simulink model "gm_parallel_lht_vnl"  (R2019b)
settings: Solver=FixedStepDiscrete  StartTime=0.0  StopTime=inf  RelTol=1e-3
undefined symbols (not defined in the file or in its folder): bt, height, nTheta, width
libraries: hdlsllib x199, simulink x27, hdlmdlgenlib x7, dspsrcs4 x1
(part 19 of 19)

== system gm_parallel_lht_vnl/Parallel LHT/Parallel LHT Kernel/Hough Kernel/Hough Kernel Symmetric Look Ahead/Look Ahead Hough/Register Bank_instance85 ==
  Data In : Inport  OutDataTypeStr=fixdt(1, 11, 0)  PortDimensions=1  SampleTime=6.66666666666667e-09
  Write Enable : Inport  Port=2  OutDataTypeStr=boolean  PortDimensions=1  SampleTime=6.66666666666667e-09
  Delay_Switch : Switch  Criteria=u2 ~= 0  Threshold=double(0)  OutDataTypeStr=fixdt(1, 11, 0)  SampleTime=6.66666666666667e-09
  Unit Delay Enabled Synchronous_lowered : Delay  DelayLength=double(1)  InitialCondition=0  SampleTime=6.66666666666667e-09
  Data Out : Outport
  wires:
  Unit Delay Enabled Synchronous_lowered/1 -> Data Out/1, Delay_Switch/3
  Data In/1 -> Delay_Switch/1
  Write Enable/1 -> Delay_Switch/2
  Delay_Switch/1 -> Unit Delay Enabled Synchronous_lowered/1

== system gm_parallel_lht_vnl/Parallel LHT/Parallel LHT Kernel/Hough Kernel/Hough Kernel Symmetric Look Ahead/Look Ahead Hough/Register Bank_instance86 ==
  Data In : Inport  OutDataTypeStr=fixdt(1, 11, 0)  PortDimensions=1  SampleTime=6.66666666666667e-09
  Write Enable : Inport  Port=2  OutDataTypeStr=boolean  PortDimensions=1  SampleTime=6.66666666666667e-09
  Delay_Switch : Switch  Criteria=u2 ~= 0  Threshold=double(0)  OutDataTypeStr=fixdt(1, 11, 0)  SampleTime=6.66666666666667e-09
  Unit Delay Enabled Synchronous_lowered : Delay  DelayLength=double(1)  InitialCondition=0  SampleTime=6.66666666666667e-09
  Data Out : Outport
  wires:
  Unit Delay Enabled Synchronous_lowered/1 -> Data Out/1, Delay_Switch/3
  Data In/1 -> Delay_Switch/1
  Write Enable/1 -> Delay_Switch/2
  Delay_Switch/1 -> Unit Delay Enabled Synchronous_lowered/1

== system gm_parallel_lht_vnl/Parallel LHT/Parallel LHT Kernel/Hough Kernel/Hough Kernel Symmetric Look Ahead/Look Ahead Hough/Register Bank_instance87 ==
  Data In : Inport  OutDataTypeStr=fixdt(1, 11, 0)  PortDimensions=1  SampleTime=6.66666666666667e-09
  Write Enable : Inport  Port=2  OutDataTypeStr=boolean  PortDimensions=1  SampleTime=6.66666666666667e-09
  Delay_Switch : Switch  Criteria=u2 ~= 0  Threshold=double(0)  OutDataTypeStr=fixdt(1, 11, 0)  SampleTime=6.66666666666667e-09
  Unit Delay Enabled Synchronous_lowered : Delay  DelayLength=double(1)  InitialCondition=0  SampleTime=6.66666666666667e-09
  Data Out : Outport
  wires:
  Unit Delay Enabled Synchronous_lowered/1 -> Data Out/1, Delay_Switch/3
  Data In/1 -> Delay_Switch/1
  Write Enable/1 -> Delay_Switch/2
  Delay_Switch/1 -> Unit Delay Enabled Synchronous_lowered/1

== system gm_parallel_lht_vnl/Parallel LHT/Parallel LHT Kernel/Hough Kernel/Hough Kernel Symmetric Look Ahead/Look Ahead Hough/Register Bank_instance88 ==
  Data In : Inport  OutDataTypeStr=fixdt(1, 11, 0)  PortDimensions=1  SampleTime=6.66666666666667e-09
  Write Enable : Inport  Port=2  OutDataTypeStr=boolean  PortDimensions=1  SampleTime=6.66666666666667e-09
  Delay_Switch : Switch  Criteria=u2 ~= 0  Threshold=double(0)  OutDataTypeStr=fixdt(1, 11, 0)  SampleTime=6.66666666666667e-09
  Unit Delay Enabled Synchronous_lowered : Delay  DelayLength=double(1)  InitialCondition=0  SampleTime=6.66666666666667e-09
  Data Out : Outport
  wires:
  Unit Delay Enabled Synchronous_lowered/1 -> Data Out/1, Delay_Switch/3
  Data In/1 -> Delay_Switch/1
  Write Enable/1 -> Delay_Switch/2
  Delay_Switch/1 -> Unit Delay Enabled Synchronous_lowered/1

== system gm_parallel_lht_vnl/Parallel LHT/Parallel LHT Kernel/Hough Kernel/Hough Kernel Symmetric Look Ahead/Look Ahead Hough/Register Bank_instance89 ==
  Data In : Inport  OutDataTypeStr=fixdt(1, 11, 0)  PortDimensions=1  SampleTime=6.66666666666667e-09
  Write Enable : Inport  Port=2  OutDataTypeStr=boolean  PortDimensions=1  SampleTime=6.66666666666667e-09
  Delay_Switch : Switch  Criteria=u2 ~= 0  Threshold=double(0)  OutDataTypeStr=fixdt(1, 11, 0)  SampleTime=6.66666666666667e-09
  Unit Delay Enabled Synchronous_lowered : Delay  DelayLength=double(1)  InitialCondition=0  SampleTime=6.66666666666667e-09
  Data Out : Outport
  wires:
  Unit Delay Enabled Synchronous_lowered/1 -> Data Out/1, Delay_Switch/3
  Data In/1 -> Delay_Switch/1
  Write Enable/1 -> Delay_Switch/2
  Delay_Switch/1 -> Unit Delay Enabled Synchronous_lowered/1

== system gm_parallel_lht_vnl/Parallel LHT/Parallel LHT Kernel/Hough Kernel/Hough Kernel Symmetric Look Ahead/Look Ahead Hough/Register Bank_instance9 ==
  Data In : Inport  OutDataTypeStr=fixdt(1, 11, 0)  PortDimensions=1  SampleTime=6.66666666666667e-09
  Write Enable : Inport  Port=2  OutDataTypeStr=boolean  PortDimensions=1  SampleTime=6.66666666666667e-09
  Delay_Switch : Switch  Criteria=u2 ~= 0  Threshold=double(0)  OutDataTypeStr=fixdt(1, 11, 0)  SampleTime=6.66666666666667e-09
  Unit Delay Enabled Synchronous_lowered : Delay  DelayLength=double(1)  InitialCondition=0  SampleTime=6.66666666666667e-09
  Data Out : Outport
  wires:
  Unit Delay Enabled Synchronous_lowered/1 -> Data Out/1, Delay_Switch/3
  Data In/1 -> Delay_Switch/1
  Write Enable/1 -> Delay_Switch/2
  Delay_Switch/1 -> Unit Delay Enabled Synchronous_lowered/1

== system gm_parallel_lht_vnl/Parallel LHT/Parallel LHT Kernel/Hough Kernel/Hough Kernel Symmetric Look Ahead/Look Ahead Hough/Register Bank_instance90 ==
  Data In : Inport  OutDataTypeStr=fixdt(1, 11, 0)  PortDimensions=1  SampleTime=6.66666666666667e-09
  Write Enable : Inport  Port=2  OutDataTypeStr=boolean  PortDimensions=1  SampleTime=6.66666666666667e-09
  Delay_Switch : Switch  Criteria=u2 ~= 0  Threshold=double(0)  OutDataTypeStr=fixdt(1, 11, 0)  SampleTime=6.66666666666667e-09
  Unit Delay Enabled Synchronous_lowered : Delay  DelayLength=double(1)  InitialCondition=0  SampleTime=6.66666666666667e-09
  Data Out : Outport
  wires:
  Unit Delay Enabled Synchronous_lowered/1 -> Data Out/1, Delay_Switch/3
  Data In/1 -> Delay_Switch/1
  Write Enable/1 -> Delay_Switch/2
  Delay_Switch/1 -> Unit Delay Enabled Synchronous_lowered/1

== system gm_parallel_lht_vnl/Parallel LHT/Parallel LHT Kernel/Hough Kernel/Hough Kernel Symmetric Look Ahead/Look Ahead Hough/Register Bank_instance91 ==
  Data In : Inport  OutDataTypeStr=fixdt(1, 11, 0)  PortDimensions=1  SampleTime=6.66666666666667e-09
  Write Enable : Inport  Port=2  OutDataTypeStr=boolean  PortDimensions=1  SampleTime=6.66666666666667e-09
  Delay_Switch : Switch  Criteria=u2 ~= 0  Threshold=double(0)  OutDataTypeStr=fixdt(1, 11, 0)  SampleTime=6.66666666666667e-09
  Unit Delay Enabled Synchronous_lowered : Delay  DelayLength=double(1)  InitialCondition=0  SampleTime=6.66666666666667e-09
  Data Out : Outport
  wires:
  Unit Delay Enabled Synchronous_lowered/1 -> Data Out/1, Delay_Switch/3
  Data In/1 -> Delay_Switch/1
  Write Enable/1 -> Delay_Switch/2
  Delay_Switch/1 -> Unit Delay Enabled Synchronous_lowered/1

== system gm_parallel_lht_vnl/Parallel LHT_vnl/Parallel LHT Accumulator/Accumulator with Switches/Accumulator/Block RAM/Simple Dual Port RAM ==
  wr_data : Inport
  wr_addr : Inport  Port=2
  wr_en : Inport  Port=3
  rd_addr : Inport  Port=4
  Simple Dual Port RAM : hdlsllib/HDL RAMs/Simple Dual Port RAM  ram_size=ceil(log2(maxRho*2))
      settings: SourceProductName=Simulink  SourceProductBaseCode=SL
  rd_data : Outport
  wires:
  Simple Dual Port RAM/1 -> rd_data/1
  rd_addr/1 -> Simple Dual Port RAM/4
  wr_en/1 -> Simple Dual Port RAM/3
  wr_addr/1 -> Simple Dual Port RAM/2
  wr_data/1 -> Simple Dual Port RAM/1

== system gm_parallel_lht_vnl/Parallel LHT_vnl/Parallel LHT Accumulator/Accumulator with Switches/Accumulator/Block RAM/Simple Dual Port RAM Generator ==
  wr_data : Inport
  wr_addr : Inport  Port=2
  wr_en : Inport  Port=3
  rd_addr : Inport  Port=4
  rd_address : hdlsllib/Logic and Bit Operations/Bit Slice  lidx=9  ridx=0
      settings: SourceProductName=Simulink  SourceProductBaseCode=SL
  simple_ram_0 : hdlsllib/HDL RAMs/Simple Dual Port RAM  ram_size=10
      settings: SourceProductName=Simulink  SourceProductBaseCode=SL
  wr_address : hdlsllib/Logic and Bit Operations/Bit Slice  lidx=9  ridx=0
      settings: SourceProductName=Simulink  SourceProductBaseCode=SL
  rd_data : Outport
  wires:
  simple_ram_0/1 -> rd_data/1
  rd_address/1 -> simple_ram_0/4
  rd_addr/1 -> rd_address/1
  wr_en/1 -> simple_ram_0/3
  wr_address/1 -> simple_ram_0/2
  wr_addr/1 -> wr_address/1
  wr_data/1 -> simple_ram_0/1

== system gm_parallel_lht_vnl/Parallel LHT_vnl/Parallel LHT Kernel/Hough Kernel/Hough Kernel Symmetric Look Ahead/Look Ahead Hough/Register Bank ==
  Data In : Inport
  Write Enable : Inport  Port=2  Partition=on  PartitionDimension=2  PartitionWidth=1  PartitionOffset=0
  For Each : ForEach  DisableCoverage=on
  Unit Delay Enabled Synchronous : hdlsllib/Discrete/Unit Delay Enabled Synchronous  InitialCondition=0.0  SampleTime=-1
      settings: SourceProductName=Simulink  SourceProductBaseCode=SL
  Data Out : Outport  ConcatenationDimension=2
  wires:
  Write Enable/1 -> Unit Delay Enabled Synchronous/2
  Unit Delay Enabled Synchronous/1 -> Data Out/1
  Data In/1 -> Unit Delay Enabled Synchronous/1

== matlab function gm_parallel_lht_vnl/Parallel LHT_vnl/Parallel LHT Accumulator/Accumulator Controller ==
  data: sof input; mode output; eof input; read output; clear output; index output; ntheta input; nrho input; valid output
function [mode, read, clear, index, valid] = fcn(sof, eof, ntheta, nrho)

IDLE = fi(0, 0, 2, 0);
VOTE = fi(1, 0, 2, 0);
READ = fi(2, 0, 2, 0);
CLEAR = fi(3, 0, 2, 0);

persistent current_state;
persistent rho_counter;
persistent theta_counter;

if isempty(current_state)
    current_state = IDLE;
end

if isempty(rho_counter)
    rho_counter = fi(0, 0, 16, 0);
end

if isempty(theta_counter)
    theta_counter = fi(0, 0, 16, 0);
end

switch current_state
    case IDLE
        rho_counter = fi(0, 0, 16, 0);
        theta_counter = fi(0, 0, 16, 0);
        
        clear = false;
        read = rho_counter;
        index = theta_counter;
        valid = false;
        
        if sof
            mode = true;
            current_state = VOTE;
        else
            mode = false;
            current_state = IDLE;
        end
        
    case VOTE
        rho_counter = fi(0, 0, 16, 0);
        theta_counter = fi(0, 0, 16, 0);
        
        mode = true;
        clear = false;
        valid = false;
        
        read = rho_counter;
        index = theta_counter;
        
        if eof
            current_state = READ;
        else
            current_state = VOTE;
        end
        
    case READ
        mode = false;
        clear = false;
        read = rho_counter;
        index = theta_counter;
        valid = true;
        
        if theta_counter >= nrho && rho_counter >= ntheta
            rho_counter = fi(0, 0, 16, 0);
            theta_counter = fi(0, 0, 16, 0);
            current_state = CLEAR;
        elseif rho_counter >= nrho
            theta_counter = fi(theta_counter + 1, 0, 16, 0);
            rho_counter = fi(0, 0, 16, 0);
            current_state = READ;
        else
            rho_counter = fi(rho_counter + 1, 0, 16, 0);
            current_state = READ;
        end
        
    case CLEAR
        mode = false;
        clear = true;
        valid = false;
        
        read = rho_counter;
        index = theta_counter;
        
        if rho_counter >= nrho
            rho_counter = fi(0, 0, 16, 0);
            theta_counter = fi(0, 0, 16, 0);
            current_state = IDLE;
        else
            rho_counter = fi(rho_counter + 1, 0, 16, 0);
            theta_counter = fi(0, 0, 16, 0);
            current_state = CLEAR;
        end
        
    otherwise
        rho_counter = fi(0, 0, 16, 0);
        theta_counter = fi(0, 0, 16, 0);
        
        mode = false;
        clear = false;
        valid = false;
        
        read = rho_counter;
        index = theta_counter;
        
        current_state = IDLE;
        
end

== matlab function gm_parallel_lht_vnl/Parallel LHT/Parallel LHT Accumulator/Accumulator Controller/Accumulator Controller ==
  data: sof input; mode output; eof input; read output; clear output; index output; ntheta input; nrho input; valid output
function [mode, read, clear, index, valid] = fcn(sof, eof, ntheta, nrho)

IDLE = fi(0, 0, 2, 0);
VOTE = fi(1, 0, 2, 0);
READ = fi(2, 0, 2, 0);
CLEAR = fi(3, 0, 2, 0);

persistent current_state;
persistent rho_counter;
persistent theta_counter;

if isempty(current_state)
    current_state = IDLE;
end

if isempty(rho_counter)
    rho_counter = fi(0, 0, 16, 0);
end

if isempty(theta_counter)
    theta_counter = fi(0, 0, 16, 0);
end

switch current_state
    case IDLE
        rho_counter = fi(0, 0, 16, 0);
        theta_counter = fi(0, 0, 16, 0);
        
        clear = false;
        read = rho_counter;
        index = theta_counter;
        valid = false;
        
        if sof
            mode = true;
            current_state = VOTE;
        else
            mode = false;
            current_state = IDLE;
        end
        
    case VOTE
        rho_counter = fi(0, 0, 16, 0);
        theta_counter = fi(0, 0, 16, 0);
        
        mode = true;
        clear = false;
        valid = false;
        
        read = rho_counter;
        index = theta_counter;
        
        if eof
            current_state = READ;
        else
            current_state = VOTE;
        end
        
    case READ
        mode = false;
        clear = false;
        read = rho_counter;
        index = theta_counter;
        valid = true;
        
        if theta_counter >= nrho && rho_counter >= ntheta
            rho_counter = fi(0, 0, 16, 0);
            theta_counter = fi(0, 0, 16, 0);
            current_state = CLEAR;
        elseif rho_counter >= nrho
            theta_counter = fi(theta_counter + 1, 0, 16, 0);
            rho_counter = fi(0, 0, 16, 0);
            current_state = READ;
        else
            rho_counter = fi(rho_counter + 1, 0, 16, 0);
            current_state = READ;
        end
        
    case CLEAR
        mode = false;
        clear = true;
        valid = false;
        
        read = rho_counter;
        index = theta_counter;
        
        if rho_counter >= nrho
            rho_counter = fi(0, 0, 16, 0);
            theta_counter = fi(0, 0, 16, 0);
            current_state = IDLE;
        else
            rho_counter = fi(rho_counter + 1, 0, 16, 0);
            theta_counter = fi(0, 0, 16, 0);
            current_state = CLEAR;
        end
        
    otherwise
        rho_counter = fi(0, 0, 16, 0);
        theta_counter = fi(0, 0, 16, 0);
        
        mode = false;
        clear = false;
        valid = false;
        
        read = rho_counter;
        index = theta_counter;
        
        current_state = IDLE;
        
end

== matlab function gm_parallel_lht_vnl/Parallel LHT/Parallel LHT Kernel/Hough Kernel/Hough Kernel Symmetric Look Ahead/Look Ahead Hough/MATLAB Function/MATLAB Function ==
  data: index output; eol input; sel output; write output; ntheta input; debug_state output
function [index, sel, write, debug_state] = fcn(eol, ntheta)

BANK = fi(1, 0, 3, 0);
WAIT = fi(2, 0, 3, 0);

persistent state;

persistent thetacounter;

if isempty(state)
    state = BANK;
end

if isempty(thetacounter)
    thetacounter = fi(0, 0, 16, 0);
end

switch state
    case BANK
        sel = false;
        write = true;
        index = thetacounter;
        debug_state = state;
        
        if thetacounter == ntheta
            thetacounter = fi(0, 0, 16, 0);
            state = WAIT;
        else
            thetacounter = fi(thetacounter + 1, 0, 16, 0);
            state = BANK;
        end
        
    case WAIT
        write = false;
        index = thetacounter;
        debug_state = state;
        
        thetacounter = fi(0, 0, 16, 0);
        
        if eol
            sel = true;
            state = BANK;
        else
            sel = false;
            state = WAIT;
        end
        
    otherwise
        thetacounter = fi(0, 0, 16, 0);
        sel = false;
        write = false;
        index = thetacounter;
        debug_state = state;
        
        state = WAIT;
        
end

== matlab function gm_parallel_lht_vnl/Parallel LHT_vnl/Parallel LHT Kernel/Hough Kernel/Hough Kernel Symmetric Look Ahead/Look Ahead Hough/MATLAB Function ==
  data: index output; eol input; sel output; write output; ntheta input; debug_state output
function [index, sel, write, debug_state] = fcn(eol, ntheta)

BANK = fi(1, 0, 3, 0);
WAIT = fi(2, 0, 3, 0);

persistent state;

persistent thetacounter;

if isempty(state)
    state = BANK;
end

if isempty(thetacounter)
    thetacounter = fi(0, 0, 16, 0);
end

switch state
    case BANK
        sel = false;
        write = true;
        index = thetacounter;
        debug_state = state;
        
        if thetacounter == ntheta
            thetacounter = fi(0, 0, 16, 0);
            state = WAIT;
        else
            thetacounter = fi(thetacounter + 1, 0, 16, 0);
            state = BANK;
        end
        
    case WAIT
        write = false;
        index = thetacounter;
        debug_state = state;
        
        thetacounter = fi(0, 0, 16, 0);
        
        if eol
            sel = true;
            state = BANK;
        else
            sel = false;
            state = WAIT;
        end
        
    otherwise
        thetacounter = fi(0, 0, 16, 0);
        sel = false;
        write = false;
        index = thetacounter;
        debug_state = state;
        
        state = WAIT;
        
end
